simulink model "Motor_Model"  (R2020b)
settings: Solver=ode45  StartTime=0.0  StopTime=10  RelTol=1e-3
settings Model: Creator=sansh  LastModifiedBy=mucah
settings DataIOCC: ReturnWorkspaceOutputs=off
settings DebuggingCC: ArithmeticOperatorsInVariantConditions=warning
settings SFSimCC: SimUseLocalCustomCode=off  CustomCodeUndefinedFunction=UseInterfaceOnly
settings RTWCC: RTWUseLocalCustomCode=off
settings CodeAppCC: StateflowObjectComments=on

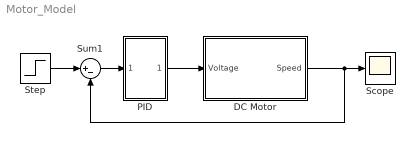
== system Motor_Model ==
  DC Motor : Subsystem
  PID : Subsystem  mask{P=20, I=0, D=20}
      mask prompts: P "Kp"; I "Ki"; D "Kd"
  Scope : Scope
  Step : Step  After=10  SampleTime=0.1
  Sum1 : Sum  Inputs=|+-
  wires:
  DC Motor/1(Speed) -> Scope/1, Sum1/2
  Step/1 -> Sum1/1
  Sum1/1 -> PID/1(In1)
  PID/1(Out1) -> DC Motor/1(Voltage)

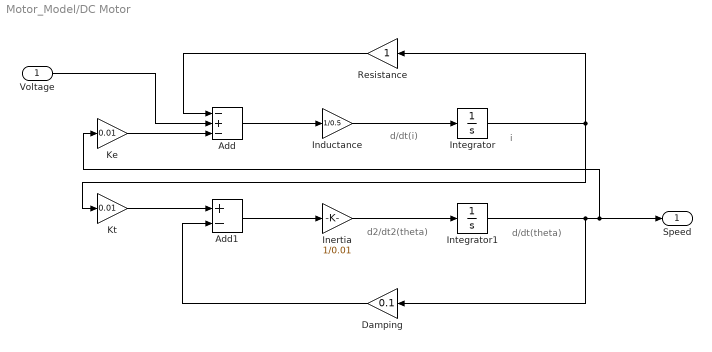
== system Motor_Model/DC Motor ==
  note: i
  note: d/dt(i)
  note: d/dt(theta)
  note: d2/dt2(theta)
  Voltage : Inport
  Add : Sum  Inputs=-+-
  Add1 : Sum  Inputs=+-
  Damping : Gain  Gain=0.1
  Inductance : Gain  Gain=1/0.5
  Inertia : Gain  Gain=1/0.01
  Integrator : Integrator
  Integrator1 : Integrator
  Ke : Gain  Gain=0.01
  Kt : Gain  Gain=0.01
  Resistance : Gain
  Speed : Outport
  wires:
  Inductance/1 -> Integrator/1
  Integrator1/1 -> Damping/1, Speed/1, Ke/1
  Inertia/1 -> Integrator1/1
  Integrator/1 -> Resistance/1, Kt/1
  Kt/1 -> Add1/1
  Voltage/1 -> Add/2
  Resistance/1 -> Add/1
  Damping/1 -> Add1/2
  Ke/1 -> Add/3
  Add/1 -> Inductance/1
  Add1/1 -> Inertia/1

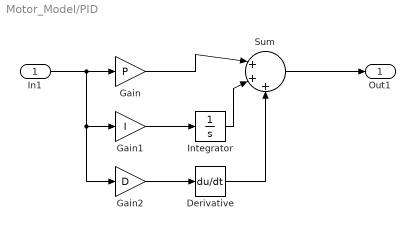
== system Motor_Model/PID ==
  In1 : Inport
  Derivative : Derivative
  Gain : Gain  Gain=P
  Gain1 : Gain  Gain=I
  Gain2 : Gain  Gain=D
  Integrator : Integrator
  Sum : Sum  Inputs=|+++
  Out1 : Outport
  wires:
  Gain/1 -> Sum/1
  In1/1 -> Gain2/1, Gain1/1, Gain/1
  Derivative/1 -> Sum/3
  Integrator/1 -> Sum/2
  Sum/1 -> Out1/1
  Gain2/1 -> Derivative/1
  Gain1/1 -> Integrator/1
